simulink model "EcoCAR3_Capstone_P2_LEA_GKN_Enerdel_TheREALone"  (R2014a)
settings: Solver=ode45  StartTime=0.0  StopTime=10.0  RelTol=1e-3
undefined symbols (not defined in the file): chas, DriverControls, EcoCAR3_Lib, eng, eng_plant_init, engine, engine_ratio, env, ENV, fd, gb, gb_ctrl_init, gb_ctrl_trs_init, max_cap, max_cell_curr, motor_ratio, motor_sync_k, motor_sync_Kd, motor_sync_Ki, motor_sync_Kp, num_cell_par, num_cell_series, veh, VEH, veh_plant_init, vpa, vpc, vpc_brake_init, whl, whl_plant_init
libraries: simulink x20
(part 2 of 3)

== system EcoCAR3_Capstone_P2_LEA_GKN_Enerdel_TheREALone/Supervisory Controller/vpc_prop_par_direct_pwr_1mot_pretx/Subsystem ==
  accel cmd : Inport
  brake cmd : Inport  Port=2
  chas_lin_spd : Inport  Port=3
  1-D Lookup Table1 : Lookup_n-D  NumberOfTableDimensions=1  BreakpointsForDimension1=whl.plant.init.trq_brake_mech.idx1_brake_cmd  Table=whl.plant.init.trq_brake_mech.map  InternalRulePriority=Speed  RndMeth=Simplest  InputSameDT=on
  Gain : Gain  Gain=-1
  Product : Product
  Switch : Switch  Criteria=u2 > Threshold
  max_possible_whl_trq : Lookup_n-D  NumberOfTableDimensions=1  BreakpointsForDimension1=vpc.prop.init.whl_trq_max.idx1_chas_lin_spd  Table=vpc.prop.init.whl_trq_max.map  InternalRulePriority=Speed  RndMeth=Simplest  InputSameDT=on
  whl_trq_dmd : Outport
  wires:
  brake cmd/1 -> Gain/1
  Gain/1 -> 1-D Lookup Table1/1
  1-D Lookup Table1/1 -> Switch/3
  Switch/1 -> whl_trq_dmd/1
  chas_lin_spd/1 -> max_possible_whl_trq/1
  accel cmd/1 -> Product/2, Switch/2
  max_possible_whl_trq/1 -> Product/1
  Product/1 -> Switch/1

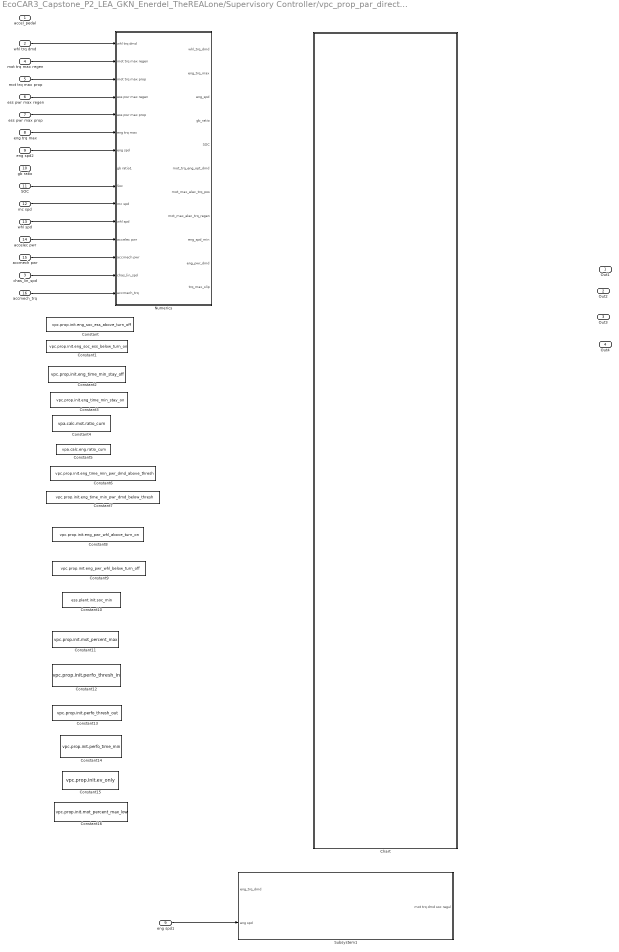
== system EcoCAR3_Capstone_P2_LEA_GKN_Enerdel_TheREALone/Supervisory Controller/vpc_prop_par_direct_pwr_1mot_pretx/control strategy ==
  accel_pedal : Inport
  whl trq dmd : Inport  Port=2
  chas_lin_spd : Inport  Port=3
  mot trq max regen : Inport  Port=4
  mot trq max prop : Inport  Port=5
  ess pwr max regen : Inport  Port=6
  ess pwr max prop : Inport  Port=7
  eng trq max : Inport  Port=8
  eng spd1 : Inport  Port=9
  gb ratio : Inport  Port=10
  SOC : Inport  Port=11
  mc spd : Inport  Port=12
  whl spd : Inport  Port=13
  accelec pwr : Inport  Port=14
  accmech pwr : Inport  Port=15
  accmech_trq : Inport  Port=16
  Chart : Stateflow chart  TreatAsAtomicUnit=on
  Constant : Constant  Value=vpc.prop.init.eng_soc_ess_above_turn_off
  Constant1 : Constant  Value=vpc.prop.init.eng_soc_ess_below_turn_on
  Constant10 : Constant  Value=ess.plant.init.soc_min
  Constant11 : Constant  Value=vpc.prop.init.mot_percent_max
  Constant12 : Constant  Value=vpc.prop.init.perfo_thresh_in
  Constant13 : Constant  Value=vpc.prop.init.perfo_thresh_out
  Constant14 : Constant  Value=vpc.prop.init.perfo_time_min
  Constant15 : Constant  Value=vpc.prop.init.ev_only
  Constant16 : Constant  Value=vpc.prop.init.mot_percent_max_low
  Constant2 : Constant  Value=vpc.prop.init.eng_time_min_stay_off
  Constant3 : Constant  Value=vpc.prop.init.eng_time_min_stay_on
  Constant4 : Constant  Value=vpa.calc.mot.ratio_cum
  Constant5 : Constant  Value=vpa.calc.eng.ratio_cum
  Constant6 : Constant  Value=vpc.prop.init.eng_time_min_pwr_dmd_above_thresh
  Constant7 : Constant  Value=vpc.prop.init.eng_time_min_pwr_dmd_below_thresh
  Constant8 : Constant  Value=vpc.prop.init.eng_pwr_whl_above_turn_on
  Constant9 : Constant  Value=vpc.prop.init.eng_pwr_whl_below_turn_off
  Numerics : Subsystem
  Subsystem1 : Subsystem
  eng spd2 : InportShadow  Port=9
  Out1 : Outport
  Out2 : Outport  Port=2
  Out3 : Outport  Port=3
  Out4 : Outport  Port=4
  wires:
  eng spd1/1 -> Subsystem1/2(eng spd)
  accmech_trq/1 -> Numerics/15(accmech_trq)
  accmech pwr/1 -> Numerics/13(accmech pwr)
  accelec pwr/1 -> Numerics/12(accelec pwr)
  whl spd/1 -> Numerics/11(whl spd)
  chas_lin_spd/1 -> Numerics/14(chas_lin_spd)
  mc spd/1 -> Numerics/10(mc spd)
  SOC/1 -> Numerics/9(Soc)
  eng spd2/1 -> Numerics/7(eng spd)
  eng trq max/1 -> Numerics/6(eng trq max)
  ess pwr max prop/1 -> Numerics/5(ess pwr max prop)
  ess pwr max regen/1 -> Numerics/4(ess pwr max regen)
  mot trq max prop/1 -> Numerics/3(mot trq max prop)
  mot trq max regen/1 -> Numerics/2(mot trq max regen)
  whl trq dmd/1 -> Numerics/1(whl trq dmd)

== system EcoCAR3_Capstone_P2_LEA_GKN_Enerdel_TheREALone/Architecture/ESS/Plant/SOC Calculation ==
  Current : Inport
  1/max_cap : Gain  Gain=1/max_cap
  Add : Sum  Inputs=-+
  Constant : Constant
  Conversion: Hours to seconds : Gain  Gain=1/3600
  Integrator : Integrator
  Saturation : Saturate  UpperLimit=1  LowerLimit=0
  SOC : Outport
  wires:
  Conversion: Hours to seconds/1 -> 1/max_cap/1
  Add/1 -> Saturation/1
  Integrator/1 -> Conversion: Hours to seconds/1
  Constant/1 -> Add/2
  Current/1 -> Integrator/1
  1/max_cap/1 -> Add/1
  Saturation/1 -> SOC/1

== system EcoCAR3_Capstone_P2_LEA_GKN_Enerdel_TheREALone/Architecture/ESS/Plant/Voltage Calculation ==
  SOC : Inport
  Current : Inport  Port=2
  1/max_cell_curr : Gain  Gain=1/max_cell_curr
  Product : Product
  Product1 : Product
  Rint : Lookup_n-D  NumberOfTableDimensions=1  BreakpointsForDimension1=[-5:5]  Table=tanh([-5:5])  InternalRulePriority=Speed  RndMeth=Simplest  InputSameDT=on
  Subtract : Sum  Inputs=+-
  Voc : Lookup_n-D  NumberOfTableDimensions=1  BreakpointsForDimension1=[-5:5]  Table=tanh([-5:5])  InternalRulePriority=Speed  RndMeth=Simplest  InputSameDT=on
  Open Circuit Voltage : Outport
  Voltage : Outport  Port=2
  Internal Resistance : Outport  Port=3
  wires:
  Current/1 -> Product1/2, 1/max_cell_curr/1
  SOC/1 -> Rint/1, Voc/1
  1/max_cell_curr/1 -> Product/2
  Rint/1 -> Product/1
  Product/1 -> Internal Resistance/1, Product1/1
  Voc/1 -> Open Circuit Voltage/1, Subtract/1
  Product1/1 -> Subtract/2
  Subtract/1 -> Voltage/1

== system EcoCAR3_Capstone_P2_LEA_GKN_Enerdel_TheREALone/Architecture/ESS/ess_controller_PI/Controller ==
  Current : Inport
  Voltage : Inport  Port=2
  SOC : Inport  Port=3
  Current1 : Inport  Port=4
  Interpolation (curr)1 : Fcn  Expr=u(3)*u(1) + u(2)*(1-u(1))
  Interpolation (curr)2 : Fcn  Expr=u(3)*u(1) + u(2)*(1-u(1))
  Mux : Mux  Inputs=3
  Mux1 : Mux  Inputs=3
  Product : Product
  Saturation : Saturate  UpperLimit=inf  LowerLimit=0
  Saturation1 : Saturate  UpperLimit=inf  LowerLimit=0
  Subsystem : Subsystem
  Subsystem1 : Subsystem
  continuous max discharge current : Lookup_n-D  NumberOfTableDimensions=1  BreakpointsForDimension1=[-5:5]  Table=tanh([-5:5])  InternalRulePriority=Speed  RndMeth=Simplest  InputSameDT=on
  continuous max power : Lookup_n-D  NumberOfTableDimensions=1  BreakpointsForDimension1=[-5:5]  Table=tanh([-5:5])  InternalRulePriority=Speed  RndMeth=Simplest  InputSameDT=on
  number of parallel : Gain
  number of parallel1 : Gain
  pulse max discharge current : Lookup_n-D  NumberOfTableDimensions=1  BreakpointsForDimension1=[-5:5]  Table=tanh([-5:5])  InternalRulePriority=Speed  RndMeth=Simplest  InputSameDT=on
  pulse max power : Lookup_n-D  NumberOfTableDimensions=1  BreakpointsForDimension1=[-5:5]  Table=tanh([-5:5])  InternalRulePriority=Speed  RndMeth=Simplest  InputSameDT=on
  total number of cells : Gain
  total number of cells1 : Gain
  power_max_prop : Outport
  current_max_prop : Outport  Port=2
  wires:
  Subsystem1/1(current ratio) -> Mux1/1
  Saturation1/1 -> Subsystem1/1(current)
  Interpolation (curr)2/1 -> current_max_prop/1
  Mux1/1 -> Interpolation (curr)2/1
  number of parallel/1 -> Mux1/2, Subsystem1/2(continuous max discharge current)
  number of parallel1/1 -> Mux1/3
  Current1/1 -> Saturation1/1
  Interpolation (curr)1/1 -> power_max_prop/1
  Mux/1 -> Interpolation (curr)1/1
  Subsystem/1(power ratio) -> Mux/1
  total number of cells1/1 -> Mux/3
  total number of cells/1 -> Subsystem/2(continuous max power), Mux/2
  Saturation/1 -> Subsystem/1(power)
  Product/1 -> Saturation/1
  Voltage/1 -> Product/2
  Current/1 -> Product/1
  continuous max power/1 -> total number of cells/1
  pulse max power/1 -> total number of cells1/1
  continuous max discharge current/1 -> number of parallel/1
  pulse max discharge current/1 -> number of parallel1/1
  SOC/1 -> pulse max discharge current/1, continuous max discharge current/1, continuous max power/1, pulse max power/1

== system EcoCAR3_Capstone_P2_LEA_GKN_Enerdel_TheREALone/Architecture/ESS/ess_controller_PI/Controller1 ==
  Current : Inport
  Voltage : Inport  Port=2
  SOC : Inport  Port=3
  Current1 : Inport  Port=4
  Interpolation (curr)1 : Fcn  Expr=u(3)*u(1) + u(2)*(1-u(1))
  Interpolation (curr)2 : Fcn  Expr=u(3)*u(1) + u(2)*(1-u(1))
  Mux : Mux  Inputs=3
  Mux1 : Mux  Inputs=3
  Product : Product
  Saturation : Saturate  UpperLimit=0  LowerLimit=-inf
  Saturation1 : Saturate  UpperLimit=0  LowerLimit=-inf
  Subsystem : Subsystem
  Subsystem1 : Subsystem
  continuous max discharge current : Lookup_n-D  NumberOfTableDimensions=1  BreakpointsForDimension1=[-5:5]  Table=tanh([-5:5])  InternalRulePriority=Speed  RndMeth=Simplest  InputSameDT=on
  continuous max power : Lookup_n-D  NumberOfTableDimensions=1  BreakpointsForDimension1=[-5:5]  Table=tanh([-5:5])  InternalRulePriority=Speed  RndMeth=Simplest  InputSameDT=on
  number of parallel : Gain
  number of parallel1 : Gain
  pulse max discharge current : Lookup_n-D  NumberOfTableDimensions=1  BreakpointsForDimension1=[-5:5]  Table=tanh([-5:5])  InternalRulePriority=Speed  RndMeth=Simplest  InputSameDT=on
  pulse max power : Lookup_n-D  NumberOfTableDimensions=1  BreakpointsForDimension1=[-5:5]  Table=tanh([-5:5])  InternalRulePriority=Speed  RndMeth=Simplest  InputSameDT=on
  total number of cells : Gain
  total number of cells1 : Gain
  power_max_reg : Outport
  current_max_reg : Outport  Port=2
  wires:
  SOC/1 -> pulse max power/1, continuous max power/1, continuous max discharge current/1, pulse max discharge current/1
  pulse max discharge current/1 -> number of parallel1/1
  continuous max discharge current/1 -> number of parallel/1
  pulse max power/1 -> total number of cells1/1
  continuous max power/1 -> total number of cells/1
  Current/1 -> Product/1
  Voltage/1 -> Product/2
  Product/1 -> Saturation/1
  Saturation/1 -> Subsystem/1(power)
  total number of cells/1 -> Mux/2, Subsystem/2(continuous max power)
  total number of cells1/1 -> Mux/3
  Subsystem/1(power ratio) -> Mux/1
  Mux/1 -> Interpolation (curr)1/1
  Interpolation (curr)1/1 -> power_max_reg/1
  Current1/1 -> Saturation1/1
  number of parallel1/1 -> Mux1/3
  number of parallel/1 -> Subsystem1/2(continuous max discharge current), Mux1/2
  Mux1/1 -> Interpolation (curr)2/1
  Interpolation (curr)2/1 -> current_max_reg/1
  Saturation1/1 -> Subsystem1/1(current)
  Subsystem1/1(current ratio) -> Mux1/1

== system EcoCAR3_Capstone_P2_LEA_GKN_Enerdel_TheREALone/Architecture/Engine/Controller/Bus In ==
  In1 : Inport
  Out1 : Outport
  wires:
  In1/1 -> Out1/1

== system EcoCAR3_Capstone_P2_LEA_GKN_Enerdel_TheREALone/Architecture/Engine/Controller/Command block  ==
  note: mux
  eng_trq_dmd : Inport
  eng_trq_mx : Inport  Port=2
  eng_trq_min : Inport  Port=3
  eng_on : Inport  Port=4
  (0,1) : Saturate  UpperLimit=1  LowerLimit=0
  Bus Creator : BusCreator  Inputs=3
  Fcn : Fcn  Expr=(u(1)-u(3))/((u(2)-u(3))+eps)*((u(2)-u(3))!=0)*(u(1)!=0)
  eng_ctrl_cmd_on_simu : Outport
  eng_ctrl_cmd_simu : Outport  Port=2
  wires:
  Fcn/1 -> (0,1)/1
  Bus Creator/1 -> Fcn/1
  eng_trq_mx/1 -> Bus Creator/2
  eng_trq_min/1 -> Bus Creator/3
  (0,1)/1 -> [eng_ctrl_cmd_simu]
  eng_on/1 -> [eng_ctrl_cmd_on_simu]
  [eng_ctrl_on_simu] -> eng_ctrl_cmd_on_simu/1
  [eng_ctrl_cmd_simu] -> eng_ctrl_cmd_simu/1
  eng_trq_dmd/1 -> Bus Creator/1

== system EcoCAR3_Capstone_P2_LEA_GKN_Enerdel_TheREALone/Architecture/Engine/Controller/Constraints Block ==
  eng_trq_dmd1 : Inport
  Hot ctt torque : Lookup_n-D  NumberOfTableDimensions=1  BreakpointsForDimension1=eng.plant.init.trq_min_hot.idx1_spd  Table=eng.plant.init.trq_min_hot.map  InternalRulePriority=Speed  RndMeth=Simplest  InputSameDT=on
  Hot wott torque : Lookup_n-D  NumberOfTableDimensions=1  BreakpointsForDimension1=eng.plant.init.trq_max_hot.idx1_spd  Table=eng.plant.init.trq_max_hot.map  InternalRulePriority=Speed  RndMeth=Simplest  InputSameDT=on
  eng_ctrl_cstr_trq_hot_max_simu : Outport
  eng_ctrl_cstr_trq_hot_min_simu : Outport  Port=2
  wires:
  [eng_ctrl_cstr_trq_hot_max_simu] -> eng_ctrl_cstr_trq_hot_max_simu/1
  [eng_ctrl_cstr_trq_hot_simu] -> eng_ctrl_cstr_trq_hot_min_simu/1
  eng_trq_dmd1/1 -> Hot ctt torque/1, Hot wott torque/1
  Hot wott torque/1 -> [eng_ctrl_cstr_trq_hot_max_simu]
  Hot ctt torque/1 -> [eng_ctrl_cstr_trq_hot_simu]

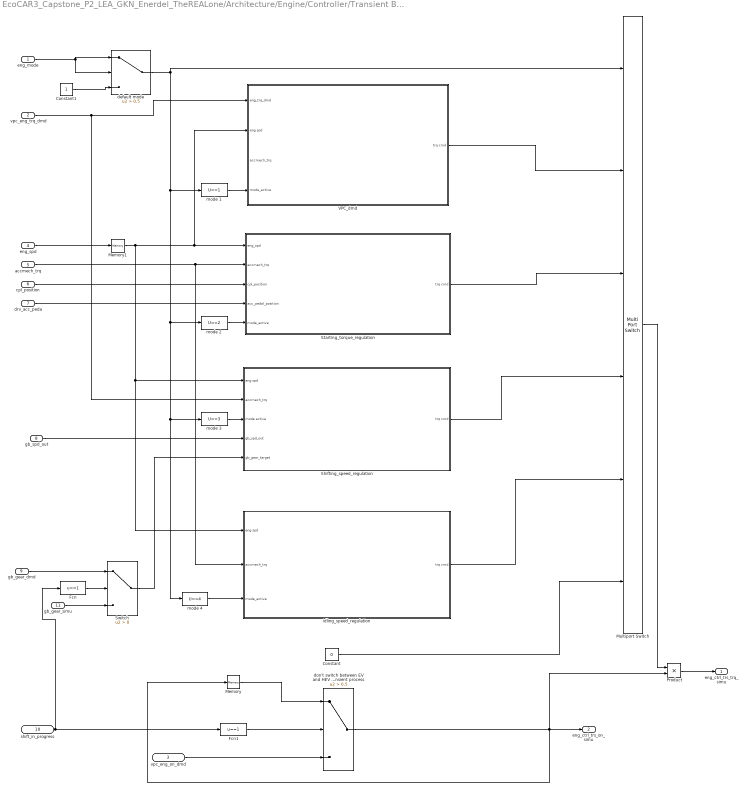
== system EcoCAR3_Capstone_P2_LEA_GKN_Enerdel_TheREALone/Architecture/Engine/Controller/Transient Block ==
  eng_mode : Inport
  vpc_eng_trq_dmd : Inport  Port=2
  vpc_eng_on_dmd : Inport  Port=3
  eng_spd : Inport  Port=4
  accmech_trq : Inport  Port=5
  cpl_position : Inport  Port=6
  drv_acc_peda : Inport  Port=7
  gb_spd_out : Inport  Port=8
  gb_gear_dmd : Inport  Port=9
  shift_in_progress : Inport  Port=10
  gb_gear_simu : Inport  Port=11
  Constant : Constant  Value=0
  Constant1 : Constant
  Fcn : Fcn  Expr=u==1
  Fcn1 : Fcn  Expr=u==1
  Memory : Memory
  Memory1 : Memory
  Multiport Switch : MultiPortSwitch  Inputs=5
  Product : Product
  Shifting_speed_regulation : Subsystem
  "Starting_torque_regulation " : Subsystem
  Switch : Switch  Criteria=u2 > Threshold
  VPC_dmd : Subsystem
  default mode : Switch  Criteria=u2 > Threshold  Threshold=0.5
  don't switch between EV and HEV mode when during transient process : Switch  Criteria=u2 > Threshold  Threshold=0.5
  idling_speed_regulation : Subsystem
  mode 1 : Fcn  Expr=U==1
  mode 2 : Fcn  Expr=U==2
  mode 3 : Fcn  Expr=U==3
  mode 4 : Fcn  Expr=U==4
  eng_ctrl_trs_trq_simu : Outport
  eng_ctrl_trs_on_simu : Outport  Port=2
  wires:
  shift_in_progress/1 -> Fcn/1, Fcn1/1
  vpc_eng_on_dmd/1 -> don't switch between EV and HEV mode when during transient process/3
  Fcn1/1 -> don't switch between EV and HEV mode when during transient process/2
  Memory/1 -> don't switch between EV and HEV mode when during transient process/1
  Product/1 -> eng_ctrl_trs_trq_simu/1
  Constant/1 -> Multiport Switch/6
  Multiport Switch/1 -> Product/1
  Constant1/1 -> default mode/3
  eng_mode/1 -> default mode/1, default mode/2
  eng_spd/1 -> Memory1/1
  vpc_eng_trq_dmd/1 -> VPC_dmd/1(eng_trq_dmd), Shifting_speed_regulation/2(accmech_trq)
  accmech_trq/1 -> "Starting_torque_regulation "/2(accmech_trq), idling_speed_regulation/2(accmech_trq)
  default mode/1 -> mode 3/1, mode 4/1, mode 2/1, mode 1/1, Multiport Switch/1
  Memory1/1 -> idling_speed_regulation/1(eng spd), Shifting_speed_regulation/1(eng spd), "Starting_torque_regulation "/1(eng_spd), VPC_dmd/2(eng spd)
  VPC_dmd/1(trq cmd) -> Multiport Switch/2
  cpl_position/1 -> "Starting_torque_regulation "/3(cpl_position)
  "Starting_torque_regulation "/1(trq cmd) -> Multiport Switch/3
  idling_speed_regulation/1(trq cmd) -> Multiport Switch/5
  drv_acc_peda/1 -> "Starting_torque_regulation "/4(acc_pedal_position)
  Shifting_speed_regulation/1(trq cmd) -> Multiport Switch/4
  don't switch between EV and HEV mode when during transient process/1 -> Product/2, eng_ctrl_trs_on_simu/1, Memory/1
  Fcn/1 -> Switch/2
  gb_gear_dmd/1 -> Switch/1
  gb_gear_simu/1 -> Switch/3
  Switch/1 -> Shifting_speed_regulation/5(gb_gear_target)
  mode 4/1 -> idling_speed_regulation/3(mode_active)
  mode 3/1 -> Shifting_speed_regulation/3(mode active)
  gb_spd_out/1 -> Shifting_speed_regulation/4(gb_spd_out)
  mode 2/1 -> "Starting_torque_regulation "/5(mode_active)
  mode 1/1 -> VPC_dmd/4(mode_active)

== system EcoCAR3_Capstone_P2_LEA_GKN_Enerdel_TheREALone/Architecture/Gearbox/Controller/Demand ==
  note: Making calculations on whether gear shifts can be made
  gb_gear : Inport
  drv_accel_dmd : Inport  Port=2
  chas_lin_spd : Inport  Port=3
  whl_spd_in : Inport  Port=4
  cpl_lock : Inport  Port=5
  eng_on : Inport  Port=6
  dv_spd_dmd : Inport  Port=7  Interpolate=off
  Bus Creator : BusCreator  Inputs=2
  Calculations : Subsystem
  Constant : Constant  Value=gb.ctrl.dmd.init.acc_below_no_timer
  Constant1 : Constant  Value=gb.ctrl.dmd.init.chas_spd_max_neutro
  Constant2 : Constant  Value=gb.plant.calc.gear_max
  Constant3 : Constant  Value=gb.ctrl.dmd.init.min_time_for_shift_dmd
  Gear Shift Logic : Stateflow chart  TreatAsAtomicUnit=on
  min = gb.plant.calc.gear_min max = gb.plant.calc.gear_max : Saturate  UpperLimit=gb.plant.calc.gear_max  LowerLimit=gb.plant.calc.gear_min
  gb_ctrl_dmd_gear_simu : Outport
  bus out : Outport  Port=2
  wires:
  chas_lin_spd/1 -> Calculations/3(chas spd)
  drv_accel_dmd/1 -> Calculations/2(drv accel dmd)
  dv_spd_dmd/1 -> Calculations/1(spd_dmd)
  min = gb.plant.calc.gear_min max = gb.plant.calc.gear_max/1 -> gb_ctrl_dmd_gear_simu/1
  eng_on/1 -> Calculations/7(eng on)
  cpl_lock/1 -> Calculations/6(cpl lock)
  gb_gear/1 -> Calculations/5(gb gear)
  whl_spd_in/1 -> Calculations/4(whl spd in)
  Bus Creator/1 -> bus out/1

== system EcoCAR3_Capstone_P2_LEA_GKN_Enerdel_TheREALone/Architecture/Gearbox/Controller/Transient ==
  vpc_eng_on_dmd : Inport
  eng_plant_on : Inport  Port=2
  eng_spd : Inport  Port=3
  cpl_spd_in : Inport  Port=4
  cpl_spd_out : Inport  Port=5
  cpl_position : Inport  Port=6
  gear_dmd : Inport  Port=7
  actual_gear : Inport  Port=8
  veh_spd : Inport  Port=9
  accel_dmd : Inport  Port=10
  Bus Creator : BusCreator  Inputs=7
  "Gearbox Transient " : Stateflow chart  TreatAsAtomicUnit=on
  accel_stop_threshold : Constant  Value=gb_ctrl_trs_init
  cpl_spd_clutching_threshold : Constant  Value=gb_ctrl_trs_init
  cpl_spd_lockup_threshold : Constant  Value=gb_ctrl_trs_init
  eng_spd_idle : Constant  Value=eng_plant_init
  sft_time : Constant  Value=gb_ctrl_init
  veh_spd_begin_stopping : Constant  Value=gb_ctrl_trs_init
  veh_spd_stop_threshold : Constant  Value=gb_ctrl_trs_init
  bus out : Outport
  wires:
  vpc_eng_on_dmd/1 -> "Gearbox Transient "/1(eng_on_dmd)
  eng_plant_on/1 -> "Gearbox Transient "/2(eng_on)
  eng_spd/1 -> "Gearbox Transient "/3(eng_spd)
  cpl_spd_in/1 -> "Gearbox Transient "/4(cpl_spd_in)
  cpl_spd_out/1 -> "Gearbox Transient "/5(cpl_spd_out)
  cpl_position/1 -> "Gearbox Transient "/6(cpl_position)
  gear_dmd/1 -> "Gearbox Transient "/7(gear_dmd)
  actual_gear/1 -> "Gearbox Transient "/8(actual_gear)
  accel_dmd/1 -> "Gearbox Transient "/9(accel_dmd)
  veh_spd/1 -> "Gearbox Transient "/10(veh_spd)
  eng_spd_idle/1 -> "Gearbox Transient "/11(eng_spd_idle)
  veh_spd_stop_threshold/1 -> "Gearbox Transient "/12(eng_stop_threshold)
  veh_spd_begin_stopping/1 -> "Gearbox Transient "/13(veh_spd_begin_stopping), "Gearbox Transient "/14(veh_spd_started)
  cpl_spd_lockup_threshold/1 -> "Gearbox Transient "/15(cpl_lockup_threshold)
  cpl_spd_clutching_threshold/1 -> "Gearbox Transient "/16(cpl_clutching_threshold)
  accel_stop_threshold/1 -> "Gearbox Transient "/17(accel_stop_threshold)
  sft_time/1 -> "Gearbox Transient "/18(shift_time)
  "Gearbox Transient "/1(eng_mode) -> Bus Creator/1  "gb_ctrl_trs_eng_mode_simu"
  "Gearbox Transient "/2(motor_mode) -> Bus Creator/2  "gb_ctrl_trs_mot_mode_simu"
  "Gearbox Transient "/3(cpl_mode) -> Bus Creator/3  "gb_ctrl_trs_cpl_mode_simuu"
  "Gearbox Transient "/4(shift_in_prog) -> Bus Creator/4  "gb_ctrl_trs_sft_in_progress_simu"
  "Gearbox Transient "/5(veh_mode) -> Bus Creator/5  "gb_ctrl_trs_veh_mode_simu"
  "Gearbox Transient "/6(gear_cmd) -> Bus Creator/6  "gb_ctrl_trs_gear_simu"
  "Gearbox Transient "/7(previous_gear) -> Bus Creator/7  "gb_ctrl_trs_previous_gear_simu"
  Bus Creator/1 -> bus out/1

== system EcoCAR3_Capstone_P2_LEA_GKN_Enerdel_TheREALone/Architecture/Motor/Controller/Motor Controller ==
  Motor Mode : Inport
  Powertrain Controller Torque DMD : Inport  Port=2
  GB Gear DMD : Inport  Port=3
  GB SPD Out : Inport  Port=4
  Coupler Torque : Inport  Port=5
  Max Positive Motor Torque : Inport  Port=6
  Max Negative Motor Torque : Inport  Port=7
  ESS Max Power : Inport  Port=8
  Motor SPD : Inport  Port=9
  Motor Temp Coeff : Inport  Port=10
  Motor Controller Command Map : Subsystem
  "Motor Controller Constraint Map " : Subsystem
  Motor Controller Transient : Subsystem
  Motor Controller CMD : Outport
  Motor Controller Transient Value : Outport  Port=2
  Motor Controller Constraint Peak Positive Torque : Outport  Port=3
  Motor Controller Constraint Continuous Positive Torque : Outport  Port=4
  Motor Controller Constraint Peak Negative Torque : Outport  Port=5
  Motor Controller Constraint Continuous Negative Torque : Outport  Port=6
  Motor Controller Constraint Temp Coeff : Outport  Port=7
  Motor Controller Constraint Max Positive Torque : Outport  Port=8
  Motor Controller Constraint Max Negative Torque : Outport  Port=9
  wires:
  Motor Controller Transient/1(Motor Controller Transient Value) -> Motor Controller Transient Value/1, Motor Controller Command Map/1(Motor Controller Transient Value)
  "Motor Controller Constraint Map "/7(Motor Controller Constraint Max Negative Torque) -> Motor Controller Constraint Max Negative Torque/1, Motor Controller Command Map/3(Motor Controller Constraint Max Negative Torque)
  "Motor Controller Constraint Map "/6(Motor Controller Constraint Max Positive Torque) -> Motor Controller Constraint Max Positive Torque/1, Motor Controller Command Map/2(Motor Controller Constraint Max Positive Torque)
  Motor Controller Command Map/1(Motor Controller CMD) -> Motor Controller CMD/1
  Motor Mode/1 -> Motor Controller Transient/1(Motor Mode)
  GB Gear DMD/1 -> Motor Controller Transient/3(GB Gear DMD)
  Coupler Torque/1 -> Motor Controller Transient/5(Coupler Torque)
  Max Negative Motor Torque/1 -> Motor Controller Transient/7(Max Negative Motor Torque)
  Motor SPD/1 -> Motor Controller Command Map/4(Motor Plant SPD Out), "Motor Controller Constraint Map "/1(Motor SPD Out), Motor Controller Transient/9(Motor SPD)
  Motor Temp Coeff/1 -> "Motor Controller Constraint Map "/2(Motor Temp Coeff)
  "Motor Controller Constraint Map "/1(Motor Controller Constraint Peak Positive Torque) -> Motor Controller Constraint Peak Positive Torque/1
  "Motor Controller Constraint Map "/2(Motor Controller Constraint Continuous Positive Torque) -> Motor Controller Constraint Continuous Positive Torque/1
  "Motor Controller Constraint Map "/3(Motor Controller Constraint Peak Negative Torque) -> Motor Controller Constraint Peak Negative Torque/1
  "Motor Controller Constraint Map "/4(Motor Controller Constraint Continuous Negative Torque) -> Motor Controller Constraint Continuous Negative Torque/1
  "Motor Controller Constraint Map "/5(Motor Controller Constraint Temp Coeff) -> Motor Controller Constraint Temp Coeff/1
  ESS Max Power/1 -> Motor Controller Transient/8(ESS Max Power)
  Max Positive Motor Torque/1 -> Motor Controller Transient/6(Max Positive Motor Torque)
  GB SPD Out/1 -> Motor Controller Transient/4(GB SPD Out)
  Powertrain Controller Torque DMD/1 -> Motor Controller Transient/2(Powertrain Controller Torque DMD)

== system EcoCAR3_Capstone_P2_LEA_GKN_Enerdel_TheREALone/Architecture/Motor/Plant/Motor ==
  Motor Speed : Inport
  Torque CMD % : Inport  Port=2
  Voltage : Inport  Port=3
  Divide : Product  Inputs=*/
  Divide1 : Product  Inputs=*/
  Memory : Memory
  Power Efficiency : Lookup_n-D  BreakpointsForDimension1=[1:3]  BreakpointsForDimension2=[1:3]  InternalRulePriority=Speed  RndMeth=Simplest  InputSameDT=on
  Product : Product
  Product1 : Product
  Product2 : Product
  Subsystem : Subsystem
  Switch : Switch  Criteria=u2 > Threshold
  Torque out : Outport
  Current : Outport  Port=2
  wires:
  Product/1 -> Product1/1, Memory/1, Torque out/1, Power Efficiency/1  "Motor Torque"
  Torque CMD %/1 -> Subsystem/2(command), Switch/2, Product/2
  Motor Speed/1 -> Product1/2, Power Efficiency/2, Subsystem/1(motor speed)
  Subsystem/1(max torque) -> Product/1
  Memory/1 -> Subsystem/3(torque)
  Voltage/1 -> Divide/2
  Divide/1 -> Current/1
  Power Efficiency/1 -> Divide1/2, Product2/1
  Product1/1 -> Divide1/1, Product2/2
  Divide1/1 -> Switch/1
  Product2/1 -> Switch/3
  Switch/1 -> Divide/1

== system EcoCAR3_Capstone_P2_LEA_GKN_Enerdel_TheREALone/Supervisory Controller/Brake/Brake ECU Torque/Divider ==
  In1 : Inport
  In2 : Inport  Port=2
  Mux : Mux  Inputs=2
  Returns 0 or 1 : Fcn  Expr=u[1]/(u[2]+(u[2]==0))*(u[2]!=0)
  Out1 : Outport
  wires:
  Returns 0 or 1/1 -> Out1/1
  In2/1 -> Mux/2
  In1/1 -> Mux/1
  Mux/1 -> Returns 0 or 1/1

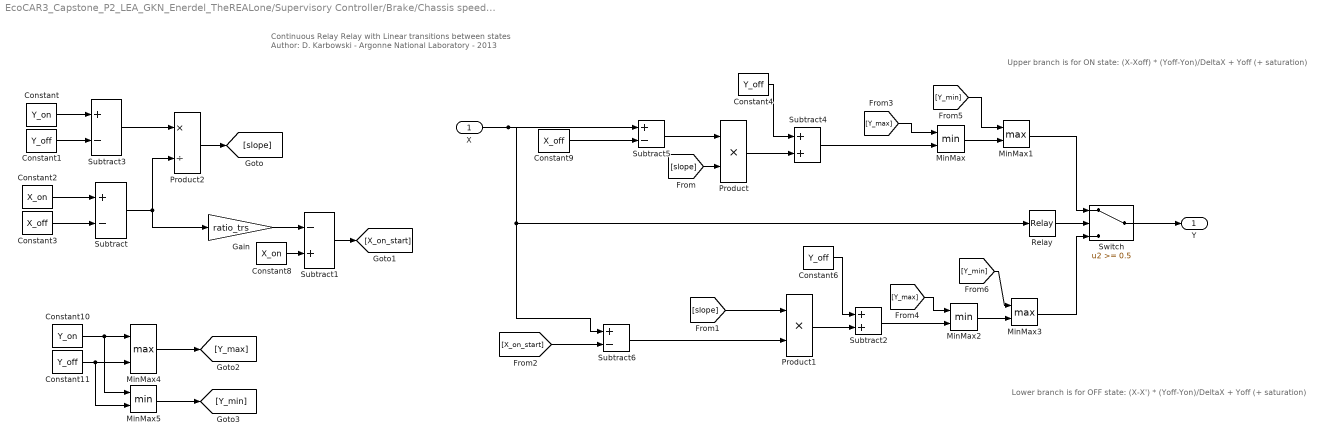
== system EcoCAR3_Capstone_P2_LEA_GKN_Enerdel_TheREALone/Supervisory Controller/Brake/Chassis speed ESS SOC limits/Continuous Relay ==
  note: Continuous Relay
      | Relay with Linear transitions between states
      | Author: D. Karbowski - Argonne National Laboratory - 2013
  note: Upper branch is for ON state: (X-Xoff) * (Yoff-Yon)/DeltaX + Yoff (+ saturation)
  note: Lower branch is for OFF state: (X-X') * (Yoff-Yon)/DeltaX + Yoff (+ saturation)
  X : Inport
  Constant : Constant  Value=Y_on
  Constant{1,4,6,11} (4 alike) : Constant  Value=Y_off
  Constant10 : Constant  Value=Y_on
  Constant2 : Constant  Value=X_on
  Constant3 : Constant  Value=X_off
  Constant8 : Constant  Value=X_on
  Constant9 : Constant  Value=X_off
  Gain : Gain  Gain=ratio_trs
  MinMax : MinMax  Inputs=2
  MinMax1 : MinMax  Function=max  Inputs=2
  MinMax2 : MinMax  Inputs=2
  MinMax3 : MinMax  Function=max  Inputs=2
  MinMax4 : MinMax  Function=max  Inputs=2
  MinMax5 : MinMax  Inputs=2
  Product : Product  RndMeth=Zero
  Product1 : Product  RndMeth=Zero
  Product2 : Product  Inputs=*/  RndMeth=Zero
  Relay : Relay  OnSwitchValue=X_on  OffSwitchValue=X_off
  Subtract{,3,5..6} (4 alike) : Sum  Inputs=+-
  Subtract1 : Sum  Inputs=-+
  Subtract2 : Sum  Inputs=2
  Subtract4 : Sum  Inputs=2
  Switch : Switch  Threshold=0.5
  Y : Outport
  wires:
  Constant2/1 -> Subtract/1
  Constant3/1 -> Subtract/2
  Constant/1 -> Subtract3/1
  Constant1/1 -> Subtract3/2
  X/1 -> Subtract5/1, Subtract6/1, Relay/1
  Product/1 -> Subtract4/2
  MinMax/1 -> MinMax1/2
  Constant4/1 -> Subtract4/1
  Relay/1 -> Switch/2
  MinMax1/1 -> Switch/1
  MinMax3/1 -> Switch/3
  Switch/1 -> Y/1
  Subtract3/1 -> Product2/1
  Subtract/1 -> Product2/2, Gain/1
  Gain/1 -> Subtract1/1
  Constant8/1 -> Subtract1/2
  Subtract5/1 -> Product/1
  Constant9/1 -> Subtract5/2
  Subtract4/1 -> MinMax/2
  Constant6/1 -> Subtract2/1
  Subtract6/1 -> Product1/2
  Product1/1 -> Subtract2/2
  Subtract2/1 -> MinMax2/2
  MinMax2/1 -> MinMax3/2
  Product2/1 -> [slope]
  Subtract1/1 -> [X_on_start]
  Constant10/1 -> MinMax4/1, MinMax5/1
  Constant11/1 -> MinMax4/2, MinMax5/2
  MinMax4/1 -> [Y_max]
  MinMax5/1 -> [Y_min]
  [slope] -> Product/2
  [slope] -> Product1/1
  [X_on_start] -> Subtract6/2
  [Y_max] -> MinMax/1
  [Y_max] -> MinMax2/1
  [Y_min] -> MinMax1/1
  [Y_min] -> MinMax3/1

== system EcoCAR3_Capstone_P2_LEA_GKN_Enerdel_TheREALone/Supervisory Controller/Brake/Chassis speed ESS SOC limits/Mechanical Regen Blending ==
  chas_spd : Inport
  Add1 : Sum  Inputs=+-
  Add2 : Sum  Inputs=+-
  Divide : Product  Inputs=*/
  Saturation1 : Saturate
  chas_spd_above_full_regen : Constant  Value=vpc_brake_init
  chas_spd_below_no_regen : Constant  Value=vpc_brake_init
  chas_spd_below_no_regen1 : Constant  Value=vpc_brake_init
  blend_factor : Outport
  wires:
  chas_spd_above_full_regen/1 -> Add1/1
  chas_spd/1 -> Add2/1
  Add2/1 -> Divide/1
  chas_spd_below_no_regen1/1 -> Add1/2
  chas_spd_below_no_regen/1 -> Add2/2
  Divide/1 -> Saturation1/1
  Add1/1 -> Divide/2
  Saturation1/1 -> blend_factor/1

== system EcoCAR3_Capstone_P2_LEA_GKN_Enerdel_TheREALone/Supervisory Controller/Brake/Gear shifting/Smooth Step Transition ==
  note: Smooth Step Transition
      | Adds a smooth transitions between at a discontinuity
      | Author: D. Karbowski - Argonne National Laboratory - 2013
  note: Normalization to [0-1]
  note: Denormalization
  note: 5-95%% of 1st order filter
  X : Inport
  X_max : Inport  Port=2
  X_min : Inport  Port=3
  1st order filter : TransferFcn  Denominator=[tau/3 1]
  Constant : Constant  Value=0.05
  Constant1 : Constant
  Fcn : Fcn  Expr=1/(1-2*u)
  MinMax : MinMax  Function=max  Inputs=2
  MinMax1 : MinMax  Inputs=2
  Product : Product  RndMeth=Zero
  Product1 : Product  Inputs=*/  RndMeth=Zero
  Product2 : Product  RndMeth=Zero
  Subtract : Sum  Inputs=-+
  Subtract1 : Sum  Inputs=+-
  Subtract2 : Sum  Inputs=+-
  Subtract3 : Sum  Inputs=-+
  Subtract4 : Sum  Inputs=2
  Out1 : Outport
  wires:
  Constant1/1 -> Subtract/2
  Subtract/1 -> MinMax1/2
  MinMax/1 -> MinMax1/1
  1st order filter/1 -> MinMax/1
  Constant/1 -> MinMax/2, Subtract/1, Subtract2/2, Fcn/1
  MinMax1/1 -> Subtract2/1
  Subtract2/1 -> Product/1
  Fcn/1 -> Product/2
  X/1 -> Subtract1/1
  Product/1 -> Product2/1
  X_min/1 -> Subtract1/2, Subtract3/1, Subtract4/2
  X_max/1 -> Subtract3/2
  Product1/1 -> 1st order filter/1
  Subtract1/1 -> Product1/1
  Subtract3/1 -> Product1/2, Product2/2
  Product2/1 -> Subtract4/1
  Subtract4/1 -> Out1/1

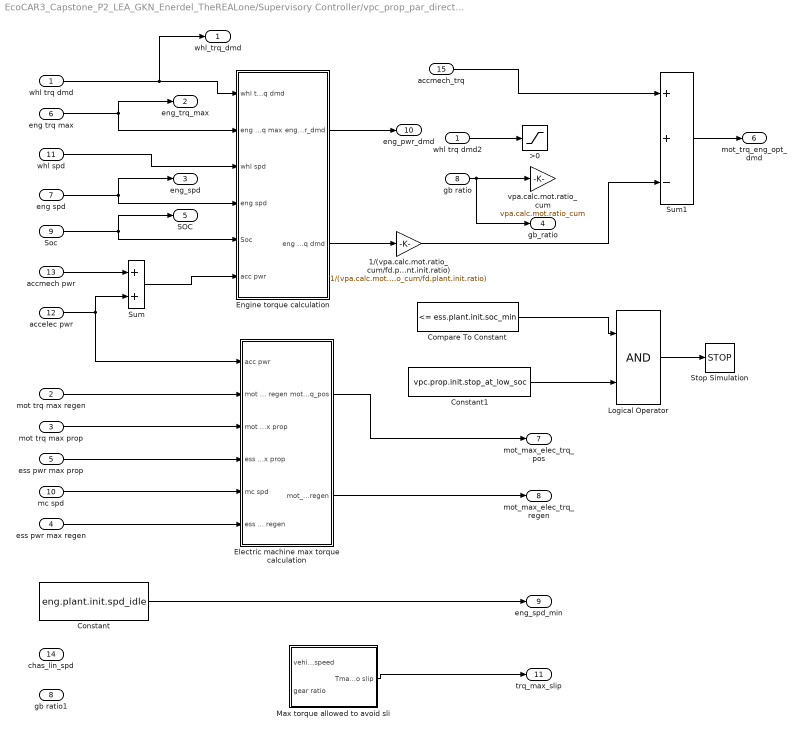
== system EcoCAR3_Capstone_P2_LEA_GKN_Enerdel_TheREALone/Supervisory Controller/vpc_prop_par_direct_pwr_1mot_pretx/control strategy/Numerics ==
  whl trq dmd : Inport
  mot trq max regen : Inport  Port=2
  mot trq max prop : Inport  Port=3
  ess pwr max regen : Inport  Port=4
  ess pwr max prop : Inport  Port=5
  eng trq max : Inport  Port=6
  eng spd : Inport  Port=7
  gb ratio1 : Inport  Port=8
  Soc : Inport  Port=9
  mc spd : Inport  Port=10
  whl spd : Inport  Port=11
  accelec pwr : Inport  Port=12
  accmech pwr : Inport  Port=13
  chas_lin_spd : Inport  Port=14
  accmech_trq : Inport  Port=15
  1/(vpa.calc.mot.ratio_cum/fd.plant.init.ratio) : Gain  Gain=1/(vpa.calc.mot.ratio_cum/fd.plant.init.ratio)
  >0 : Saturate  UpperLimit=inf  LowerLimit=0
  Compare To Constant : simulink/Logic and Bit Operations/Compare To Constant  relop=<=  const=ess.plant.init.soc_min  OutDataTypeStr=uint8  ZeroCross=off
  Constant : Constant  Value=eng.plant.init.spd_idle
  Constant1 : Constant  Value=vpc.prop.init.stop_at_low_soc
  Electric machine max torque calculation : Subsystem
  Engine torque calculation : Subsystem
  Logical Operator : Logic  AllPortsSameDT=off  OutDataTypeStr=boolean
  Max torque allowed to avoid sli : Subsystem
  Stop Simulation : Stop
  Sum : Sum
  Sum1 : Sum  Inputs=++-
  gb ratio : InportShadow  Port=8
  vpa.calc.mot.ratio_cum : Gain  Gain=vpa.calc.mot.ratio_cum
  whl trq dmd2 : InportShadow
  whl_trq_dmd : Outport
  eng_trq_max : Outport  Port=2
  eng_spd : Outport  Port=3
  gb_ratio : Outport  Port=4
  SOC : Outport  Port=5
  mot_trq_eng_opt_dmd : Outport  Port=6
  mot_max_elec_trq_pos : Outport  Port=7
  mot_max_elec_trq_regen : Outport  Port=8
  eng_spd_min : Outport  Port=9
  eng_pwr_dmd : Outport  Port=10
  trq_max_slip : Outport  Port=11
  wires:
  whl trq dmd/1 -> Engine torque calculation/1(whl trq dmd), whl_trq_dmd/1
  accmech pwr/1 -> Sum/1
  accelec pwr/1 -> Electric machine max torque calculation/1(acc pwr), Sum/2
  eng trq max/1 -> Engine torque calculation/2(eng trq max), eng_trq_max/1
  eng spd/1 -> eng_spd/1, Engine torque calculation/4(eng spd)
  Soc/1 -> SOC/1, Engine torque calculation/5(Soc)
  accmech_trq/1 -> Sum1/1
  Sum1/1 -> mot_trq_eng_opt_dmd/1
  Logical Operator/1 -> Stop Simulation/1
  Compare To Constant/1 -> Logical Operator/1
  Constant1/1 -> Logical Operator/2
  whl trq dmd2/1 -> >0/1
  gb ratio/1 -> gb_ratio/1, vpa.calc.mot.ratio_cum/1
  1/(vpa.calc.mot.ratio_cum/fd.plant.init.ratio)/1 -> Sum1/3
  Constant/1 -> eng_spd_min/1
  Max torque allowed to avoid sli/1(Tmax for no slip) -> trq_max_slip/1
  Engine torque calculation/1(eng_pwr_dmd) -> eng_pwr_dmd/1
  Engine torque calculation/2(eng trq dmd) -> 1/(vpa.calc.mot.ratio_cum/fd.plant.init.ratio)/1
  whl spd/1 -> Engine torque calculation/3(whl spd)
  Sum/1 -> Engine torque calculation/6(acc pwr)
  ess pwr max regen/1 -> Electric machine max torque calculation/6(ess pwr max regen)
  mc spd/1 -> Electric machine max torque calculation/5(mc spd)
  ess pwr max prop/1 -> Electric machine max torque calculation/4(ess pwr max prop)
  mot trq max prop/1 -> Electric machine max torque calculation/3(mot trq max prop)
  mot trq max regen/1 -> Electric machine max torque calculation/2(mot trq max regen)
  Electric machine max torque calculation/2(mot_max_elec_trq_regen) -> mot_max_elec_trq_regen/1
  Electric machine max torque calculation/1(mot_max_elec_trq_pos) -> mot_max_elec_trq_pos/1

== system EcoCAR3_Capstone_P2_LEA_GKN_Enerdel_TheREALone/Supervisory Controller/vpc_prop_par_direct_pwr_1mot_pretx/control strategy/Subsystem1 ==
  eng_trq_dmd : Inport
  eng spd : Inport  Port=2
  Engine inverse hot maximum efficiency curve : Lookup_n-D  NumberOfTableDimensions=1  BreakpointsForDimension1=eng.plant.calc.trq_max_hot_mo.map  Table=eng.plant.calc.trq_max_hot_mo.idx1_spd  InternalRulePriority=Speed  RndMeth=Simplest  InputSameDT=on
  Memory : Memory
  Sum : Sum  Inputs=+-
  eng spd > idle spd : Saturate
  vpc.prop.init.mot_kp : Gain  Gain=vpc.prop.init.mot_kp
  mot trq dmd soc regul : Outport
  wires:
  vpc.prop.init.mot_kp/1 -> mot trq dmd soc regul/1
  Sum/1 -> vpc.prop.init.mot_kp/1
  eng spd/1 -> Sum/2
  eng_trq_dmd/1 -> Memory/1
  eng spd > idle spd/1 -> Sum/1
  Engine inverse hot maximum efficiency curve/1 -> eng spd > idle spd/1
  Memory/1 -> Engine inverse hot maximum efficiency curve/1

== system EcoCAR3_Capstone_P2_LEA_GKN_Enerdel_TheREALone/Architecture/ESS/ess_controller_PI/Controller/Subsystem ==
  power : Inport
  continuous max power : Inport  Port=2
  Add : Sum  Inputs=-+
  Divide : Product  Inputs=*/
  Integrator : Integrator
  Ki_power : Gain
  Saturation : Saturate  UpperLimit=1  LowerLimit=0
  power ratio : Outport
  wires:
  Integrator/1 -> Saturation/1
  Saturation/1 -> power ratio/1
  Ki_power/1 -> Integrator/1
  Divide/1 -> Ki_power/1
  Add/1 -> Divide/1
  continuous max power/1 -> Add/2, Divide/2
  power/1 -> Add/1

== system EcoCAR3_Capstone_P2_LEA_GKN_Enerdel_TheREALone/Architecture/ESS/ess_controller_PI/Controller/Subsystem1 ==
  current : Inport
  continuous max discharge current : Inport  Port=2
  Add : Sum  Inputs=-+
  Divide : Product  Inputs=*/
  Integrator : Integrator
  Ki current : Gain
  Saturation : Saturate  UpperLimit=1  LowerLimit=0
  current ratio : Outport
  wires:
  Saturation/1 -> current ratio/1
  Integrator/1 -> Saturation/1
  Ki current/1 -> Integrator/1
  Divide/1 -> Ki current/1
  Add/1 -> Divide/1
  continuous max discharge current/1 -> Add/2, Divide/2
  current/1 -> Add/1

== system EcoCAR3_Capstone_P2_LEA_GKN_Enerdel_TheREALone/Architecture/ESS/ess_controller_PI/Controller1/Subsystem ==
  power : Inport
  continuous max power : Inport  Port=2
  Add : Sum  Inputs=-+
  Divide : Product  Inputs=*/
  Integrator : Integrator
  Ki_power : Gain
  Saturation : Saturate  UpperLimit=1  LowerLimit=0
  power ratio : Outport
  wires:
  power/1 -> Add/1
  continuous max power/1 -> Add/2, Divide/2
  Add/1 -> Divide/1
  Divide/1 -> Ki_power/1
  Ki_power/1 -> Integrator/1
  Saturation/1 -> power ratio/1
  Integrator/1 -> Saturation/1

== system EcoCAR3_Capstone_P2_LEA_GKN_Enerdel_TheREALone/Architecture/ESS/ess_controller_PI/Controller1/Subsystem1 ==
  current : Inport
  continuous max discharge current : Inport  Port=2
  Add : Sum  Inputs=-+
  Divide : Product  Inputs=*/
  Integrator : Integrator
  Ki current : Gain
  Saturation : Saturate  UpperLimit=1  LowerLimit=0
  current ratio : Outport
  wires:
  current/1 -> Add/1
  continuous max discharge current/1 -> Divide/2, Add/2
  Add/1 -> Divide/1
  Divide/1 -> Ki current/1
  Ki current/1 -> Integrator/1
  Integrator/1 -> Saturation/1
  Saturation/1 -> current ratio/1

== system EcoCAR3_Capstone_P2_LEA_GKN_Enerdel_TheREALone/Architecture/Engine/Controller/Transient Block/Shifting_speed_regulation ==
  eng spd : Inport
  accmech_trq : Inport  Port=2
  mode active : Inport  Port=3
  gb_spd_out : Inport  Port=4
  gb_gear_target : Inport  Port=5
  Add : Sum  Inputs=+-
  Derivative3 : Derivative
  Gain : Gain  Gain=eng.ctrl.trs.init.shifting_k
  Integrator3 : Integrator  ExternalReset=either
  MinMax : MinMax  Function=max  Inputs=2
  Product2 : Product  RndMeth=Zero
  Saturation : Saturate  UpperLimit=150  LowerLimit=-150
  Subtract3 : Sum
  Subtract4 : Sum  Inputs=+++
  eng.plant.init.spd_idle : Constant  Value=eng.plant.init.spd_idle+20
  gear ratio table1 : Lookup  InputValues=gb.plant.init.ratio.idx1_gear  Table=gb.plant.init.ratio.map  SaturateOnIntegerOverflow=on
  kd4 : Gain  Gain=eng.ctrl.trs.init.shifting_kd
  ki4 : Gain  Gain=eng.ctrl.trs.init.shifting_ki
  kp4 : Gain  Gain=eng.ctrl.trs.init.shifting_kp
  trq cmd : Outport
  wires:
  Subtract4/1 -> Gain/1
  ki4/1 -> Integrator3/1
  mode active/1 -> Integrator3/2
  kp4/1 -> Subtract4/1
  Integrator3/1 -> Subtract4/2
  Gain/1 -> Subtract3/2
  Add/1 -> kp4/1, kd4/1, ki4/1
  gear ratio table1/1 -> Product2/1
  gb_gear_target/1 -> gear ratio table1/1
  kd4/1 -> Derivative3/1
  accmech_trq/1 -> Subtract3/1
  eng spd/1 -> Add/2
  Derivative3/1 -> Saturation/1
  Saturation/1 -> Subtract4/3
  Subtract3/1 -> trq cmd/1
  gb_spd_out/1 -> Product2/2
  Product2/1 -> MinMax/2
  MinMax/1 -> Add/1
  eng.plant.init.spd_idle/1 -> MinMax/1

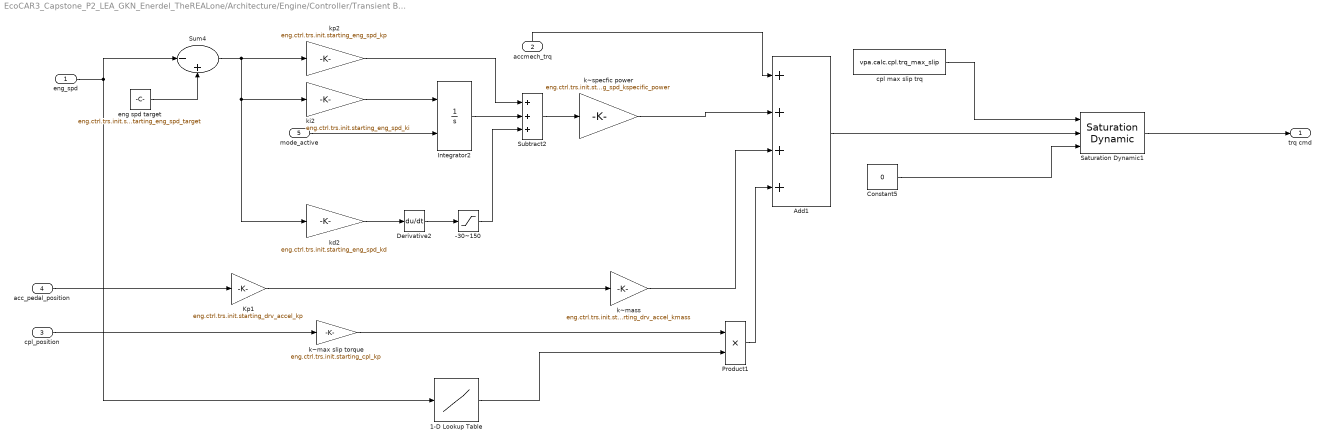
== system EcoCAR3_Capstone_P2_LEA_GKN_Enerdel_TheREALone/Architecture/Engine/Controller/Transient Block/Starting_torque_regulation  ==
  eng_spd : Inport
  accmech_trq : Inport  Port=2
  cpl_position : Inport  Port=3
  acc_pedal_position : Inport  Port=4
  mode_active : Inport  Port=5
  -30~150 : Saturate  UpperLimit=150  LowerLimit=-30
  1-D Lookup Table : Lookup_n-D  NumberOfTableDimensions=1  BreakpointsForDimension1=[0.5;1;1.5;2;2.5;3]*eng.plant.init.spd_idle  Table=[1;1;0.8;0.2;0.1;0.1]  InternalRulePriority=Speed  RndMeth=Simplest  InputSameDT=on
  Add1 : Sum  Inputs=++++
  Constant5 : Constant  Value=0
  Derivative2 : Derivative
  Integrator2 : Integrator  ExternalReset=rising
  Kp1 : Gain  Gain=eng.ctrl.trs.init.starting_drv_accel_kp
  Product1 : Product  RndMeth=Zero
  Saturation Dynamic1 : simulink/Discontinuities/Saturation Dynamic  OutMin=[]  OutMax=[]  OutDataTypeStr=Inherit: Same as second input  OutDataType=sfix(16)  OutScaling=2^-10  DoSatur=off
  Subtract2 : Sum  Inputs=+++
  Sum4 : Sum  Inputs=|-+  SaturateOnIntegerOverflow=on  InputSameDT=on  OutDataTypeStr=Inherit: Same as first input
  cpl max slip trq : Constant  Value=vpa.calc.cpl.trq_max_slip
  eng spd target : Constant  Value=eng.ctrl.trs.init.starting_eng_spd_target
  kd2 : Gain  Gain=eng.ctrl.trs.init.starting_eng_spd_kd
  ki2 : Gain  Gain=eng.ctrl.trs.init.starting_eng_spd_ki
  kp2 : Gain  Gain=eng.ctrl.trs.init.starting_eng_spd_kp
  k~mass : Gain  Gain=eng.ctrl.trs.init.starting_drv_accel_kmass
  k~max slip torque : Gain  Gain=eng.ctrl.trs.init.starting_cpl_kp
  k~specfic power : Gain  Gain=eng.ctrl.trs.init.starting_eng_spd_kspecific_power
  trq cmd : Outport
  wires:
  Product1/1 -> Add1/4
  k~max slip torque/1 -> Product1/1
  1-D Lookup Table/1 -> Product1/2
  Saturation Dynamic1/1 -> trq cmd/1
  Constant5/1 -> Saturation Dynamic1/3
  k~mass/1 -> Add1/3
  acc_pedal_position/1 -> Kp1/1
  -30~150/1 -> Subtract2/3
  Add1/1 -> Saturation Dynamic1/2
  cpl_position/1 -> k~max slip torque/1
  Kp1/1 -> k~mass/1
  kd2/1 -> Derivative2/1
  Derivative2/1 -> -30~150/1
  Sum4/1 -> kd2/1, ki2/1, kp2/1
  mode_active/1 -> Integrator2/2
  Integrator2/1 -> Subtract2/2
  kp2/1 -> Subtract2/1
  eng spd target/1 -> Sum4/2
  ki2/1 -> Integrator2/1
  Subtract2/1 -> k~specfic power/1
  k~specfic power/1 -> Add1/2
  cpl max slip trq/1 -> Saturation Dynamic1/1
  eng_spd/1 -> 1-D Lookup Table/1, Sum4/1
  accmech_trq/1 -> Add1/1

== system EcoCAR3_Capstone_P2_LEA_GKN_Enerdel_TheREALone/Architecture/Engine/Controller/Transient Block/VPC_dmd ==
  eng_trq_dmd : Inport
  eng spd : Inport  Port=2
  accmech_trq : Inport  Port=3
  mode_active : Inport  Port=4
  Derivative : Derivative
  Integrator : Integrator  ExternalReset=either
  MinMax : MinMax  Function=max  Inputs=2
  Subtract : Sum  Inputs=+++
  Sum : Sum  Inputs=+-|
  Sum1 : Sum  Inputs=++|
  eng.plant.init.spd_idle : Constant  Value=eng.plant.init.spd_idle
  k : Gain  Gain=eng.ctrl.trs.idiling_k
  kd : Gain  Gain=eng.ctrl.trs.init.idling_kd
  ki : Gain  Gain=eng.ctrl.trs.init.idling_ki
  kp : Gain  Gain=eng.ctrl.trs.init.idling_kp
  trq cmd : Outport
  wires:
  accmech_trq/1 -> Sum1/1
  eng.plant.init.spd_idle/1 -> Sum/1
  Sum/1 -> kd/1, ki/1, kp/1
  ki/1 -> Integrator/1
  Integrator/1 -> Subtract/2
  kp/1 -> Subtract/1
  Subtract/1 -> k/1
  Derivative/1 -> Subtract/3
  kd/1 -> Derivative/1
  mode_active/1 -> Integrator/2
  k/1 -> Sum1/2
  Sum1/1 -> MinMax/1
  MinMax/1 -> trq cmd/1
  eng spd/1 -> Sum/2
  eng_trq_dmd/1 -> MinMax/2

== system EcoCAR3_Capstone_P2_LEA_GKN_Enerdel_TheREALone/Architecture/Engine/Controller/Transient Block/idling_speed_regulation ==
  eng spd : Inport
  accmech_trq : Inport  Port=2
  mode_active : Inport  Port=3
  Constant3 : Constant  Value=eng.plant.init.spd_idle*1.05
  Derivative1 : Derivative
  Integrator1 : Integrator  ExternalReset=either
  Subtract1 : Sum  Inputs=+++
  Sum2 : Sum  Inputs=+-|
  Sum3 : Sum  Inputs=++|
  k1 : Gain  Gain=eng.ctrl.trs.init.idling_k
  kd1 : Gain  Gain=eng.ctrl.trs.init.idling_kd
  ki1 : Gain  Gain=eng.ctrl.trs.init.idling_ki
  kp1 : Gain  Gain=eng.ctrl.trs.init.idling_kp
  trq cmd : Outport
  wires:
  Constant3/1 -> Sum2/1
  Sum2/1 -> kd1/1, ki1/1, kp1/1
  ki1/1 -> Integrator1/1
  Integrator1/1 -> Subtract1/2
  kp1/1 -> Subtract1/1
  Subtract1/1 -> k1/1
  Derivative1/1 -> Subtract1/3
  kd1/1 -> Derivative1/1
  mode_active/1 -> Integrator1/2
  k1/1 -> Sum3/2
  Sum3/1 -> trq cmd/1
  accmech_trq/1 -> Sum3/1
  eng spd/1 -> Sum2/2

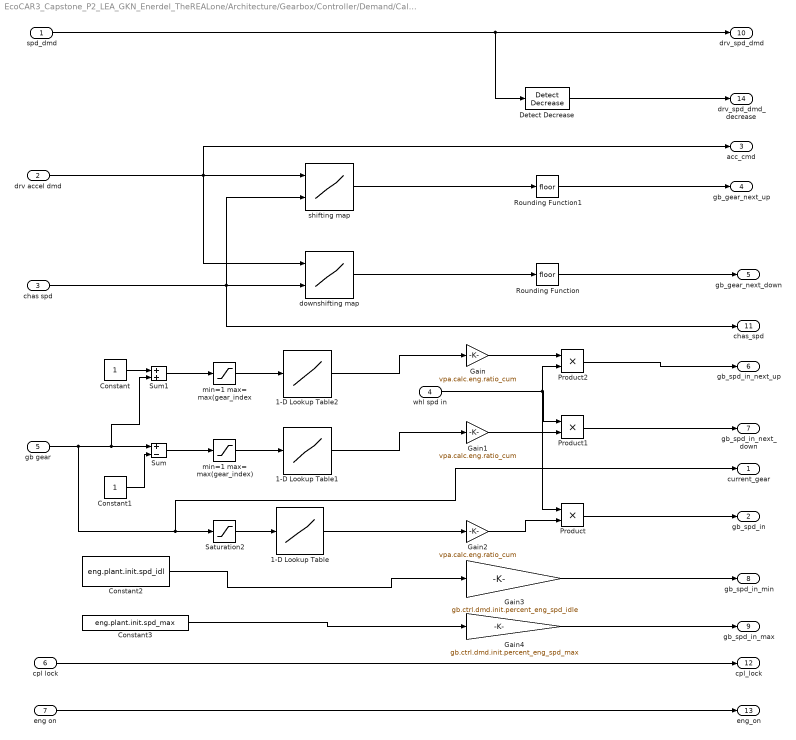
== system EcoCAR3_Capstone_P2_LEA_GKN_Enerdel_TheREALone/Architecture/Gearbox/Controller/Demand/Calculations ==
  spd_dmd : Inport
  drv accel dmd : Inport  Port=2
  chas spd : Inport  Port=3
  whl spd in : Inport  Port=4
  gb gear : Inport  Port=5
  cpl lock : Inport  Port=6
  eng on : Inport  Port=7
  1-D Lookup Table : Lookup_n-D  NumberOfTableDimensions=1  BreakpointsForDimension1=gb.plant.init.ratio.idx1_gear  Table=gb.plant.init.ratio.map  InternalRulePriority=Speed  RndMeth=Simplest  InputSameDT=on
  1-D Lookup Table1 : Lookup_n-D  NumberOfTableDimensions=1  BreakpointsForDimension1=gb.plant.init.ratio.idx1_gear  Table=gb.plant.init.ratio.map  InternalRulePriority=Speed  RndMeth=Simplest  InputSameDT=on
  1-D Lookup Table2 : Lookup_n-D  NumberOfTableDimensions=1  BreakpointsForDimension1=gb.plant.init.ratio.idx1_gear  Table=gb.plant.init.ratio.map  InternalRulePriority=Speed  RndMeth=Simplest  InputSameDT=on
  Constant : Constant
  Constant1 : Constant
  Constant2 : Constant  Value=eng.plant.init.spd_idl
  Constant3 : Constant  Value=eng.plant.init.spd_max
  Detect Decrease : simulink/Logic and Bit Operations/Detect Decrease  vinit=0.0  InputProcessing=Inherited  OutDataTypeStr=boolean
  Gain : Gain  Gain=vpa.calc.eng.ratio_cum
  Gain1 : Gain  Gain=vpa.calc.eng.ratio_cum
  Gain2 : Gain  Gain=vpa.calc.eng.ratio_cum
  Gain3 : Gain  Gain=gb.ctrl.dmd.init.percent_eng_spd_idle
  Gain4 : Gain  Gain=gb.ctrl.dmd.init.percent_eng_spd_max
  Product : Product
  Product1 : Product
  Product2 : Product
  Rounding Function : Rounding
  Rounding Function1 : Rounding
  Saturation2 : Saturate  UpperLimit=max(gb.plant.init.ratio.idx1_gear)  LowerLimit=1
  Sum : Sum  Inputs=+-
  Sum1 : Sum
  downshifting map : Lookup_n-D  BreakpointsForDimension1=gb.ctrl.dmd.init.gear_dnshift.idx1_lin_accel  BreakpointsForDimension2=gb.ctrl.dmd.init.gear_dnshift.idx2_chas_lin_spd  Table=gb.ctrl.dmd.init.gear_dnshift.map  InternalRulePriority=Speed  RndMeth=Simplest  InputSameDT=on
  min=1 max= max(gear_index : Saturate  UpperLimit=max(gb.plant.init.ratio.idx1_gear)  LowerLimit=1
  min=1 max= max(gear_index) : Saturate  UpperLimit=max(gb.plant.init.ratio.idx1_gear)  LowerLimit=1
  shifting map : Lookup_n-D  BreakpointsForDimension1=gb.ctrl.dmd.init.gear_upshift.idx1_lin_accel  BreakpointsForDimension2=gb.ctrl.dmd.init.gear_upshift.idx2_chas_lin_spd  Table=gb.ctrl.dmd.init.gear_upshift.map  InternalRulePriority=Speed  RndMeth=Simplest  InputSameDT=on
  current_gear : Outport
  gb_spd_in : Outport  Port=2
  acc_cmd : Outport  Port=3
  gb_gear_next_up : Outport  Port=4
  gb_gear_next_down : Outport  Port=5
  gb_spd_in_next_up : Outport  Port=6
  gb_spd_in_next_down : Outport  Port=7
  gb_spd_in_min : Outport  Port=8
  gb_spd_in_max : Outport  Port=9
  drv_spd_dmd : Outport  Port=10
  chas_spd : Outport  Port=11
  cpl_lock : Outport  Port=12
  eng_on : Outport  Port=13
  drv_spd_dmd_decrease : Outport  Port=14
  wires:
  eng on/1 -> eng_on/1
  cpl lock/1 -> cpl_lock/1
  Constant3/1 -> Gain4/1
  Gain4/1 -> gb_spd_in_max/1
  Constant2/1 -> Gain3/1
  Gain3/1 -> gb_spd_in_min/1
  Detect Decrease/1 -> drv_spd_dmd_decrease/1
  shifting map/1 -> Rounding Function1/1
  Rounding Function1/1 -> gb_gear_next_up/1
  downshifting map/1 -> Rounding Function/1
  Rounding Function/1 -> gb_gear_next_down/1
  1-D Lookup Table2/1 -> Gain/1
  Gain/1 -> Product2/1
  min=1 max= max(gear_index/1 -> 1-D Lookup Table2/1
  1-D Lookup Table1/1 -> Gain1/1
  1-D Lookup Table/1 -> Gain2/1
  Gain2/1 -> Product/2
  Gain1/1 -> Product1/2
  Constant/1 -> Sum1/1
  Sum1/1 -> min=1 max= max(gear_index/1
  Sum/1 -> min=1 max= max(gear_index)/1
  Saturation2/1 -> 1-D Lookup Table/1
  spd_dmd/1 -> Detect Decrease/1, drv_spd_dmd/1
  drv accel dmd/1 -> acc_cmd/1, downshifting map/1, shifting map/1
  chas spd/1 -> shifting map/2, chas_spd/1, downshifting map/2
  Constant1/1 -> Sum/2
  gb gear/1 -> current_gear/1, Saturation2/1, Sum1/2, Sum/1
  Product2/1 -> gb_spd_in_next_up/1
  Product1/1 -> gb_spd_in_next_down/1
  Product/1 -> gb_spd_in/1
  whl spd in/1 -> Product/1, Product1/1, Product2/2
  min=1 max= max(gear_index)/1 -> 1-D Lookup Table1/1

== system EcoCAR3_Capstone_P2_LEA_GKN_Enerdel_TheREALone/Architecture/Motor/Controller/Motor Controller/Motor Controller Command Map ==
  Motor Controller Transient Value : Inport
  Motor Controller Constraint Max Positive Torque : Inport  Port=2
  Motor Controller Constraint Max Negative Torque : Inport  Port=3
  Motor Plant SPD Out : Inport  Port=4
  Abs : Abs
  Abs1 : Abs
  Abs2 : Abs
  Fcn : Fcn  Expr=(u>=0)-(u<0)
  Product : Product
  Product1 : Product
  Saturation : Saturate  UpperLimit=1  LowerLimit=-1
  Subsystem : Subsystem
  Switch : Switch  Criteria=u2 > Threshold
  Motor Controller CMD : Outport
  wires:
  Motor Controller Transient Value/1 -> Product/1, Abs/1
  Motor Controller Constraint Max Positive Torque/1 -> Abs1/1
  Motor Controller Constraint Max Negative Torque/1 -> Abs2/1
  Motor Plant SPD Out/1 -> Product/2
  Abs1/1 -> Switch/1
  Abs2/1 -> Switch/3
  Product/1 -> Fcn/1, Switch/2
  Fcn/1 -> Product1/1
  Product1/1 -> Motor Controller CMD/1
  Switch/1 -> Subsystem/2(In2)
  Abs/1 -> Subsystem/1(In1)
  Subsystem/1(Out1) -> Saturation/1
  Saturation/1 -> Product1/2

== system EcoCAR3_Capstone_P2_LEA_GKN_Enerdel_TheREALone/Architecture/Motor/Controller/Motor Controller/Motor Controller Constraint Map  ==
  Motor SPD Out : Inport
  Motor Temp Coeff : Inport  Port=2
  Continuous Torque Lookup Table : Lookup_n-D  NumberOfTableDimensions=1  BreakpointsForDimension1=[-5:5]  Table=tanh([-5:5])  InternalRulePriority=Speed  RndMeth=Simplest  InputSameDT=on
  Continuous Regen Torque Lookup Table : Lookup_n-D  NumberOfTableDimensions=1  BreakpointsForDimension1=[-5:5]  Table=tanh([-5:5])  InternalRulePriority=Speed  RndMeth=Simplest  InputSameDT=on
  Fcn : Fcn  Expr=u[3]*(u[2] - u[1]) + u[1]
  Fcn1 : Fcn  Expr=u[3]*(u[2] - u[1]) + u[1]
  Mux : Mux  Inputs=3
  Mux1 : Mux  Inputs=3
  Peak Torque Lookup Table : Lookup_n-D  NumberOfTableDimensions=1  BreakpointsForDimension1=[-5:5]  Table=tanh([-5:5])  InternalRulePriority=Speed  RndMeth=Simplest  InputSameDT=on
  Peak Regen Torque Lookup Table : Lookup_n-D  NumberOfTableDimensions=1  BreakpointsForDimension1=[-5:5]  Table=tanh([-5:5])  InternalRulePriority=Speed  RndMeth=Simplest  InputSameDT=on
  Motor Controller Constraint Peak Positive Torque : Outport
  Motor Controller Constraint Continuous Positive Torque : Outport  Port=2
  Motor Controller Constraint Peak Negative Torque : Outport  Port=3
  Motor Controller Constraint Continuous Negative Torque : Outport  Port=4
  Motor Controller Constraint Temp Coeff : Outport  Port=5
  Motor Controller Constraint Max Positive Torque : Outport  Port=6
  Motor Controller Constraint Max Negative Torque : Outport  Port=7
  wires:
  Peak Torque Lookup Table/1 -> Motor Controller Constraint Peak Positive Torque/1, Mux/1
  Continuous Torque Lookup Table/1 -> Motor Controller Constraint Continuous Positive Torque/1, Mux/2
  Motor Temp Coeff/1 -> Mux/3, Motor Controller Constraint Temp Coeff/1, Mux1/3
  Motor SPD Out/1 -> Peak Regen Torque Lookup Table/1, Continuous Regen Torque Lookup Table/1, Continuous Torque Lookup Table/1, Peak Torque Lookup Table/1
  Peak Regen Torque Lookup Table/1 -> Motor Controller Constraint Peak Negative Torque/1, Mux1/1
  Continuous Regen Torque Lookup Table/1 -> Motor Controller Constraint Continuous Negative Torque/1, Mux1/2
  Mux/1 -> Fcn/1
  Mux1/1 -> Fcn1/1
  Fcn/1 -> Motor Controller Constraint Max Positive Torque/1
  Fcn1/1 -> Motor Controller Constraint Max Negative Torque/1
